simulink model "ECE_317_final"  (R2021a)
settings: Solver=VariableStepAuto  StartTime=0.0  StopTime=20  RelTol=1e-3
settings Model: Creator=sansh  LastModifiedBy=joshuahorejs
settings SolverCC: AlgebraicLoopSolver=TrustRegion
settings DataIOCC: ReturnWorkspaceOutputs=off
settings DebuggingCC: SFMachineParentedDataDiag=warning  ArithmeticOperatorsInVariantConditions=warning
settings SFSimCC: SimUseLocalCustomCode=off  CustomCodeUndefinedFunction=UseInterfaceOnly
settings RTWCC: RTWUseLocalCustomCode=off
settings CodeAppCC: StateflowObjectComments=on

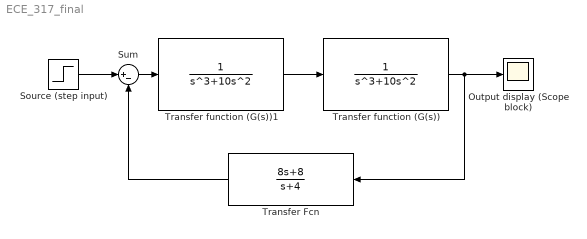
== system ECE_317_final ==
  Output display (Scope block) : Scope
  Source (step input) : Step  SampleTime=0
  Sum : Sum  Inputs=|+-
  Transfer Fcn : TransferFcn  Numerator=[8 8]  Denominator=[1 4]
  Transfer function (G(s)) : TransferFcn  Numerator=[1 ]  Denominator=[1 10 0 0]  ContinuousStateAttributes='H'
  Transfer function (G(s))1 : TransferFcn  Numerator=[1 ]  Denominator=[1 10 0 0]  ContinuousStateAttributes='H'
  wires:
  Source (step input)/1 -> Sum/1
  Transfer function (G(s))/1 -> Transfer Fcn/1, Output display (Scope block)/1
  Transfer Fcn/1 -> Sum/2
  Sum/1 -> Transfer function (G(s))1/1
  Transfer function (G(s))1/1 -> Transfer function (G(s))/1
